simulink model "model"  (Simulink 7.8)
settings: Solver=ode3  StartTime=0.0  StopTime=10.0  FixedStep=Ts  RelTol=1e-3
values from neighbouring files (symbols this model uses):
  g = 9.8065    [kostas_malakies.mat]    (also in kostas_malakies2.mat; load_PMModel.m = 9.81; main_last.m; matlab.mat)
  mass = 0.66    [kostas_malakies.mat]    (also in kostas_malakies2.mat; load_PMModel.m = 0.687; main_last.m)
  Ts = 0.02    [kostas_malakies.mat]    (also in kostas_malakies2.mat; main.m; main_last.m; matlab.mat = 0.08)
  x0 = 0    [kostas_malakies.mat]    (also in kostas_malakies2.mat; main.m; main_last.m; matlab.mat = [0 0 -1 0])
  y0 = 0    [kostas_malakies.mat]    (also in kostas_malakies2.mat; main.m; main_last.m; matlab.mat = [0 0 -1 0])
  yaw0 = 0    [kostas_malakies.mat]    (also in kostas_malakies2.mat; main.m; main_last.m; matlab.mat = -0.0873)
  z0 = 0    [kostas_malakies.mat]    (also in kostas_malakies2.mat; main.m; main_last.m; matlab.mat = [-1 0])
libraries: Hqaud_model_LIB_SI x4
settings Model: Creator=burrimi  LastModifiedBy=burrimi
settings DataIOCC: SaveOutput=off  SignalLogging=off  DSMLogging=off  SaveTime=off
settings OptimizationCC: OptimizeModelRefInitCode=on  LifeSpan=1  SimCompilerOptimization=On
settings RTWCC: SystemTargetFile=ert.tlc  TemplateMakefile=ert_default_tmf  Description=Embedded Coder  ProcessScript=ert_make_rtw_hook  CustomHeaderCode="#include \"math.h\""  TargetLang=C++  RTWCompilerOptimization=On
settings CodeAppCC: IgnoreCustomStorageClasses=off
settings ERTTargetCC: MultiwordLength=2048  GenerateSampleERTMain=on  SupportContinuousTime=on  ERTCustomFileTemplate=example_file_process.tlc  ConvertIfToSwitch=off  SuppressUnreachableDefaultCases=off

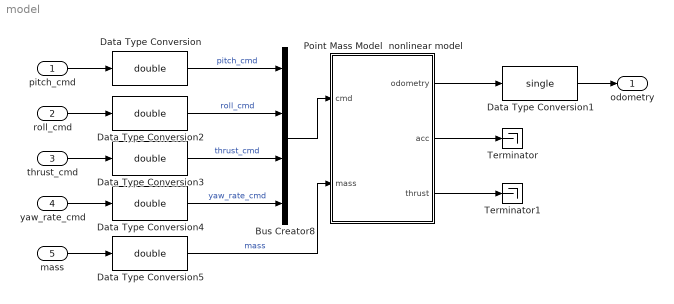
== system model ==
  pitch_cmd : Inport  OutDataTypeStr=single  PortDimensions=1  SampleTime=Ts
  roll_cmd : Inport  Port=2  OutDataTypeStr=single  PortDimensions=1  SampleTime=Ts
  thrust_cmd : Inport  Port=3  OutDataTypeStr=single  PortDimensions=1  SampleTime=Ts
  yaw_rate_cmd : Inport  Port=4  OutDataTypeStr=single  PortDimensions=1  SampleTime=Ts
  mass : Inport  Port=5  OutDataTypeStr=single
  Bus Creator8 : BusCreator
  Data Type Conversion{,2..5} (5 alike) : DataTypeConversion  OutDataTypeStr=double
  Data Type Conversion1 : DataTypeConversion  OutDataTypeStr=single
  Point Mass Model  nonlinear model : Subsystem  AncestorBlock="Hqaud_model_LIB_SI/Point Mass Model  nonlinear model"
  Terminator : Terminator
  Terminator1 : Terminator
  odometry : Outport  SampleTime=Ts
  wires:
  pitch_cmd/1 -> Data Type Conversion/1
  roll_cmd/1 -> Data Type Conversion2/1
  thrust_cmd/1 -> Data Type Conversion3/1
  yaw_rate_cmd/1 -> Data Type Conversion4/1
  Bus Creator8/1 -> Point Mass Model  nonlinear model/1(cmd)
  Point Mass Model  nonlinear model/1(odometry) -> Data Type Conversion1/1
  Point Mass Model  nonlinear model/3("thrust   ") -> Terminator1/1
  Point Mass Model  nonlinear model/2(acc) -> Terminator/1
  Data Type Conversion/1 -> Bus Creator8/1  "pitch_cmd"
  Data Type Conversion2/1 -> Bus Creator8/2  "roll_cmd"
  Data Type Conversion3/1 -> Bus Creator8/3  "thrust_cmd"
  Data Type Conversion4/1 -> Bus Creator8/4  "yaw_rate_cmd"
  Data Type Conversion1/1 -> odometry/1
  mass/1 -> Data Type Conversion5/1
  Data Type Conversion5/1 -> Point Mass Model  nonlinear model/2(mass)  "mass"

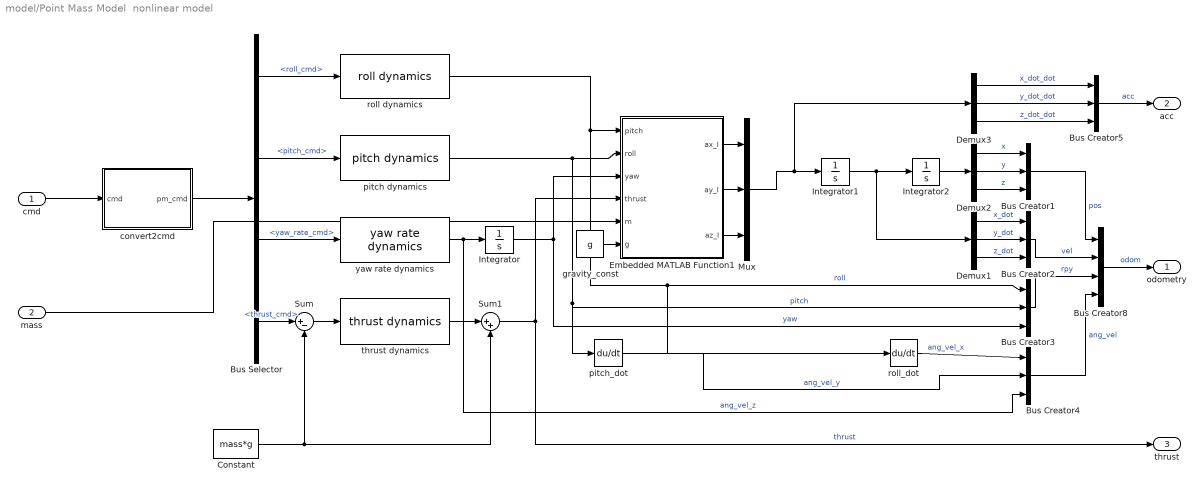
== system model/Point Mass Model  nonlinear model ==
  cmd : Inport
  mass : Inport  Port=2
  Bus Creator{1..5} (5 alike) : BusCreator  Inputs=3
  Bus Creator8 : BusCreator
  Bus Selector : BusSelector  OutputSignals=roll_cmd,pitch_cmd,yaw_rate_cmd,thrust_cmd
  Constant : Constant  Value=mass*g
  Demux1 : Demux  Outputs=3
  Demux2 : Demux  Outputs=3
  Demux3 : Demux  Outputs=3
  Embedded MATLAB Function1 : MATLAB Function  AncestorBlock=|  TreatAsAtomicUnit=on
      | Hqaud_model_LIB_SI/Newton's second law
      |  /Embedded
      | MATLAB Function1
  Integrator : Integrator  InitialCondition=yaw0
  Integrator1 : Integrator
  Integrator2 : Integrator  InitialCondition=[x0;y0;z0]
  Mux : Mux  Inputs=3
  Sum : Sum  Inputs=|+-
  Sum1 : Sum  Inputs=|++
  convert2cmd : Subsystem
  gravity_const : Constant  Value=g
  "pitch dynamics  " : Hqaud_model_LIB_SI/pitch dynamics  
  pitch_dot : Derivative
  roll dynamics : Hqaud_model_LIB_SI/roll dynamics
  roll_dot : Derivative
  "thrust dynamics  " : Hqaud_model_LIB_SI/thrust dynamics  
  "yaw rate dynamics  " : Hqaud_model_LIB_SI/yaw rate dynamics  
  odometry : Outport
  acc : Outport  Port=2
  "thrust   " : Outport  Port=3  PortDimensions=1
  wires:
  convert2cmd/1(pm_cmd) -> Bus Selector/1
  Bus Selector/1 -> roll dynamics/1  "<roll_cmd>"
  "yaw rate dynamics  "/1 -> Integrator/1, Bus Creator4/3  "ang_vel_z"
  Integrator/1 -> Bus Creator3/3, Embedded MATLAB Function1/3(yaw)  "yaw"
  "thrust dynamics  "/1 -> Sum1/1
  "pitch dynamics  "/1 -> Bus Creator3/2, pitch_dot/1, Embedded MATLAB Function1/2(roll)  "pitch"
  roll dynamics/1 -> Bus Creator3/1, roll_dot/1, Embedded MATLAB Function1/1(pitch)  "roll"
  Mux/1 -> Integrator1/1, Demux3/1
  Integrator1/1 -> Integrator2/1, Demux1/1
  Integrator2/1 -> Demux2/1
  Demux2/2 -> Bus Creator1/2  "y"
  Constant/1 -> Sum/2, Sum1/2
  Sum/1 -> "thrust dynamics  "/1
  Bus Selector/4 -> Sum/1  "<thrust_cmd>"
  cmd/1 -> convert2cmd/1(cmd)
  Bus Selector/2 -> "pitch dynamics  "/1  "<pitch_cmd>"
  Bus Selector/3 -> "yaw rate dynamics  "/1  "<yaw_rate_cmd>"
  Bus Creator4/1 -> Bus Creator8/4  "ang_vel"
  Bus Creator3/1 -> Bus Creator8/3  "rpy"
  Bus Creator2/1 -> Bus Creator8/2  "vel"
  Bus Creator1/1 -> Bus Creator8/1  "pos"
  Bus Creator8/1 -> odometry/1  "odom"
  Demux2/3 -> Bus Creator1/3  "z"
  Demux2/1 -> Bus Creator1/1  "x"
  Demux1/1 -> Bus Creator2/1  "x_dot"
  Demux1/2 -> Bus Creator2/2  "y_dot"
  Demux1/3 -> Bus Creator2/3  "z_dot"
  Bus Creator5/1 -> acc/1  "acc"
  Demux3/1 -> Bus Creator5/1  "x_dot_dot"
  Demux3/2 -> Bus Creator5/2  "y_dot_dot"
  Demux3/3 -> Bus Creator5/3  "z_dot_dot"
  Sum1/1 -> "thrust   "/1, Embedded MATLAB Function1/4(thrust)  "thrust"
  roll_dot/1 -> Bus Creator4/1  "ang_vel_x"
  pitch_dot/1 -> Bus Creator4/2  "ang_vel_y"
  gravity_const/1 -> Embedded MATLAB Function1/6(g)
  mass/1 -> Embedded MATLAB Function1/5(m)
  Embedded MATLAB Function1/2(ay_I) -> Mux/2
  Embedded MATLAB Function1/1(ax_I) -> Mux/1
  Embedded MATLAB Function1/3(az_I) -> Mux/3

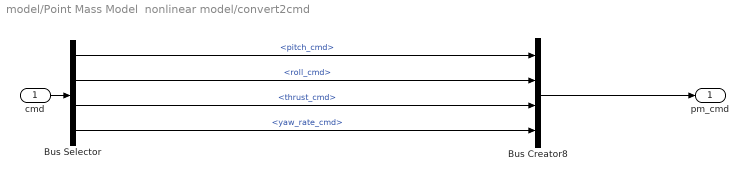
== system model/Point Mass Model  nonlinear model/convert2cmd ==
  cmd : Inport
  Bus Creator8 : BusCreator
  Bus Selector : BusSelector  OutputSignals=pitch_cmd,roll_cmd,thrust_cmd,yaw_rate_cmd
  pm_cmd : Outport
  wires:
  Bus Selector/3 -> Bus Creator8/3  "<thrust_cmd>"
  Bus Selector/4 -> Bus Creator8/4  "<yaw_rate_cmd>"
  Bus Selector/2 -> Bus Creator8/2  "<roll_cmd>"
  Bus Selector/1 -> Bus Creator8/1  "<pitch_cmd>"
  cmd/1 -> Bus Selector/1
  Bus Creator8/1 -> pm_cmd/1

== matlab function Point Mass Model nonlinear model/Embedded MATLAB Function1 ==
  data: pitch input double; ax_I output double; roll input double; yaw input double; thrust input double; m input double; g input double; ay_I output double; az_I output double
function [ax_I, ay_I, az_I] = fcn(pitch, roll, yaw, thrust, m, g)
%#eml

acc = -thrust/m*[ cos(yaw)*sin(pitch)*cos(roll)+sin(yaw)*sin(roll);...
                sin(yaw)*sin(pitch)*cos(roll)-cos(yaw)*sin(roll);...
                cos(pitch)*cos(roll)]...
             +[ 0; 0; g ];
         
ax_I = acc(1);
ay_I = acc(2);
az_I = acc(3);
